simulink model "Analog_DSSS_GC"  (Simulink 7.5)
settings: Solver=ode45  SolverMode=SingleTasking  StartTime=0.0  StopTime=50.0  RelTol=1e-3
values from neighbouring files (symbols this model uses):
  Amp = Simulink.Parameter    [Analog_DSSS_GC_saveas.m]    (also in Analog_DSSS_WH_saveas.m)
  FreqBase = Simulink.Parameter    [Analog_DSSS_GC_saveas.m]    (also in Analog_DSSS_WH_saveas.m)
  FreqCode = Simulink.Parameter    [Analog_DSSS_GC_saveas.m]    (also in Analog_DSSS_WH_saveas.m)
  Phs = Simulink.Parameter    [Analog_DSSS_GC_saveas.m]    (also in Analog_DSSS_WH_saveas.m)
libraries: dsparch4 x4, commseqgen2 x4, commutil2 x4, dspsnks4 x1
settings Model: Creator=rooki  LastModifiedBy=rooki  CovMetricSettings=dwe  CovHtmlReporting=off  covSaveCumulativeToWorkspaceVar=off  CovSaveSingleToWorkspaceVar=off  CovExternalEMLEnable=on
settings DataIOCC: LimitDataPoints=off  SaveFormat=StructureWithTime
settings OptimizationCC: ExpressionDepthLimit=128
settings DebuggingCC: UnderspecifiedInitializationDetection=Simplified  MergeDetectMultiDrivingBlocksExec=error  SolverPrmCheckMsg=none  FcnCallInpInsideContextMsg=Enable All  StateNameClashWarn=none
settings HardwareCC: ProdIntDivRoundTo=Zero  ProdEndianess=LittleEndian  ProdHWDeviceType=Specified
settings CodeAppCC: CustomSymbolStrType=$N$R$M_T
settings GRTTargetCC: TargetFunctionLibrary=C99 (ISO)  GeneratePreprocessorConditionals=Use local settings

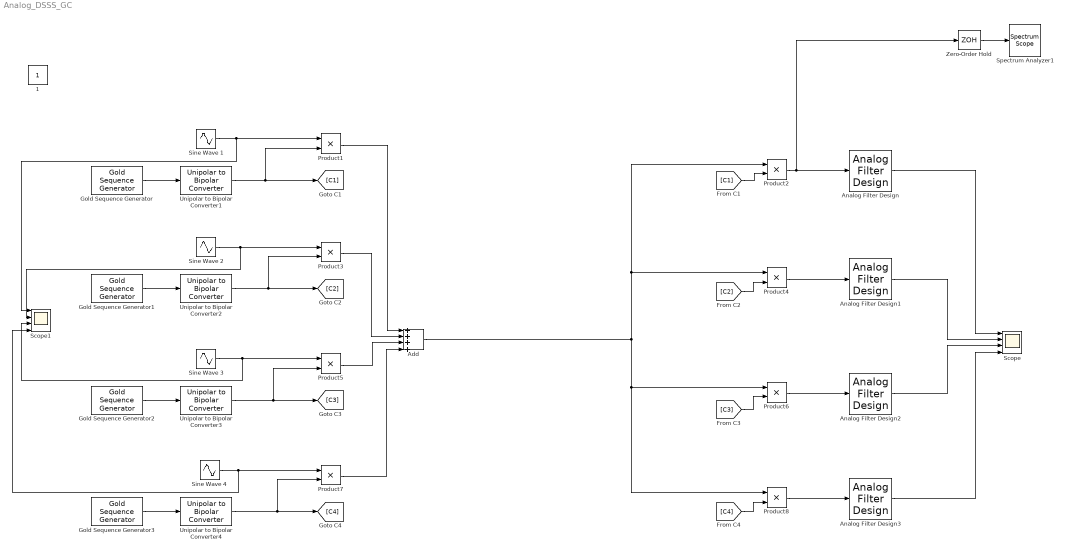
== system Analog_DSSS_GC ==
  Add : Sum  Inputs=++++
  Analog Filter Design{,1..3} (4 alike) : dsparch4/Analog Filter Design  method=Butterworth  filttype=Lowpass  N=8  Wlo=2  Whi=80  Rp=2  Rs=40
  Gold Sequence Generator : commseqgen2/Gold Sequence Generator  genPoly1="[1  0  1  1]"  iniState1=[0 0 1]  genPoly2="[1  1  0  1]"  iniState2=[0 0 1]  index=0  shift=0  Ts=FreqCode  sampPerFrame=1  reset=off  outDataType=double  frameBased=off
  Gold Sequence Generator1 : commseqgen2/Gold Sequence Generator  genPoly1="[1  0  1  1]"  iniState1=[0 0 1]  genPoly2="[1  1  0  1]"  iniState2=[0 1 0]  index=0  shift=0  Ts=FreqCode  sampPerFrame=1  reset=off  outDataType=double  frameBased=off
  Gold Sequence Generator2 : commseqgen2/Gold Sequence Generator  genPoly1="[1  0  1  1]"  iniState1=[0 0 1]  genPoly2="[1  1  0  1]"  iniState2=[0 1 1]  index=0  shift=0  Ts=FreqCode  sampPerFrame=1  reset=off  outDataType=double  frameBased=off
  Gold Sequence Generator3 : commseqgen2/Gold Sequence Generator  genPoly1="[1  0  1  1]"  iniState1=[0 0 1]  genPoly2="[1  1  0  1]"  iniState2=[1 0 0]  index=0  shift=0  Ts=FreqCode  sampPerFrame=1  reset=off  outDataType=double  frameBased=off
  Product{1..8} (8 alike) : Product
  Scope : Scope  NumInputPorts=4
      settings: TimeRange=auto  MaxDataPoints=5000  SaveToWorkspace=off  SaveName=ScopeData  YMin=-2.41765~-5~-5~-5  YMax=2.46012~5~5~5  SampleTime=-1
  Scope1 : Scope  NumInputPorts=4
      settings: TimeRange=auto  MaxDataPoints=5000  SaveToWorkspace=off  YMin=-2.49986~-5~-5~-5  YMax=2.49998~5~5~5  SampleTime=-1
  Sine Wave 1 : Sin  Amplitude=Amp(1)  Frequency=FreqBase  Phase=Phs(1)  SampleTime=0
  Sine Wave 2 : Sin  Amplitude=Amp(2)  Frequency=FreqBase  Phase=Phs(2)  SampleTime=0
  Sine Wave 3 : Sin  Amplitude=Amp(3)  Frequency=FreqBase  Phase=Phs(3)  SampleTime=0
  Sine Wave 4 : Sin  Amplitude=Amp(4)  Frequency=FreqBase  Phase=Phs(4)  SampleTime=0
  Spectrum Analyzer1 : dspsnks4/Spectrum Scope  YUnits=dBm  numAvg=1  wintypeSpecScope=Hann  RsSpecScope=50  betaSpecScope=5  XRange=Two-sided  AxisGrid=on  AxisLegend=off  Memory=off  inpFftLenInherit=on  FFTlength=1024  XLimit=Auto  XMin=0  XMax=1  UseBuffer=on  BufferSize=3075  Overlap=0  FigPos="[71.66667      14.33333           800           450]"  winsampSpecScope=Symmetric  XDisplay=0
      settings: YMin=-216.86824849143756  YMax=49.923531275391788
  Unipolar to Bipolar Converter{1..4} (4 alike) : commutil2/Unipolar to Bipolar Converter  M=2  polarity=Positive  dataType=Inherit via internal rule
  Zero-Order Hold : ZeroOrderHold  SampleTime=-1
  1 : Constant  IOType=siggen
  wires:
  Unipolar to Bipolar Converter1/1 -> Product1/2, [C1]
  Zero-Order Hold/1 -> Spectrum Analyzer1/1
  Unipolar to Bipolar Converter2/1 -> [C2], Product3/2
  Product1/1 -> Add/1
  Product3/1 -> Add/2
  Product2/1 -> Zero-Order Hold/1, Analog Filter Design/1
  Analog Filter Design/1 -> Scope/1
  Product4/1 -> Analog Filter Design1/1
  Analog Filter Design1/1 -> Scope/2
  Product5/1 -> Add/3
  Unipolar to Bipolar Converter3/1 -> [C3], Product5/2
  Product6/1 -> Analog Filter Design2/1
  Analog Filter Design2/1 -> Scope/3
  Sine Wave 1/1 -> Scope1/1, Product1/1
  Product8/1 -> Analog Filter Design3/1
  Product7/1 -> Add/4
  Unipolar to Bipolar Converter4/1 -> [C4], Product7/2
  Analog Filter Design3/1 -> Scope/4
  Sine Wave 2/1 -> Scope1/2, Product3/1
  Sine Wave 3/1 -> Scope1/3, Product5/1
  Sine Wave 4/1 -> Scope1/4, Product7/1
  [C1] -> Product2/2
  [C2] -> Product4/2
  [C3] -> Product6/2
  [C4] -> Product8/2
  Gold Sequence Generator/1 -> Unipolar to Bipolar Converter1/1
  Gold Sequence Generator1/1 -> Unipolar to Bipolar Converter2/1
  Gold Sequence Generator2/1 -> Unipolar to Bipolar Converter3/1
  Gold Sequence Generator3/1 -> Unipolar to Bipolar Converter4/1
  Add/1 -> Product8/1, Product6/1, Product4/1, Product2/1
